simulink model "ControlLineal"  (R2024a)
settings: Solver=ode4  StartTime=0.0  StopTime=20  FixedStep=.01  MinStep=.01  RelTol=1e-3
settings Model: Creator=YTLATELPO  LastModifiedBy=alegaco
settings RTWCC: GPUComputeCapability=3.5

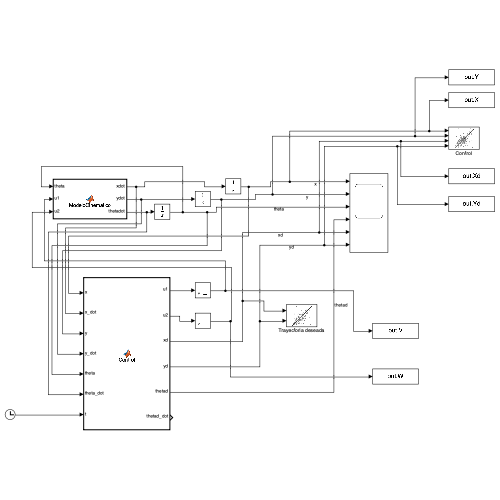
[thumbnail: Simulink's stored preview of the top-level diagram]
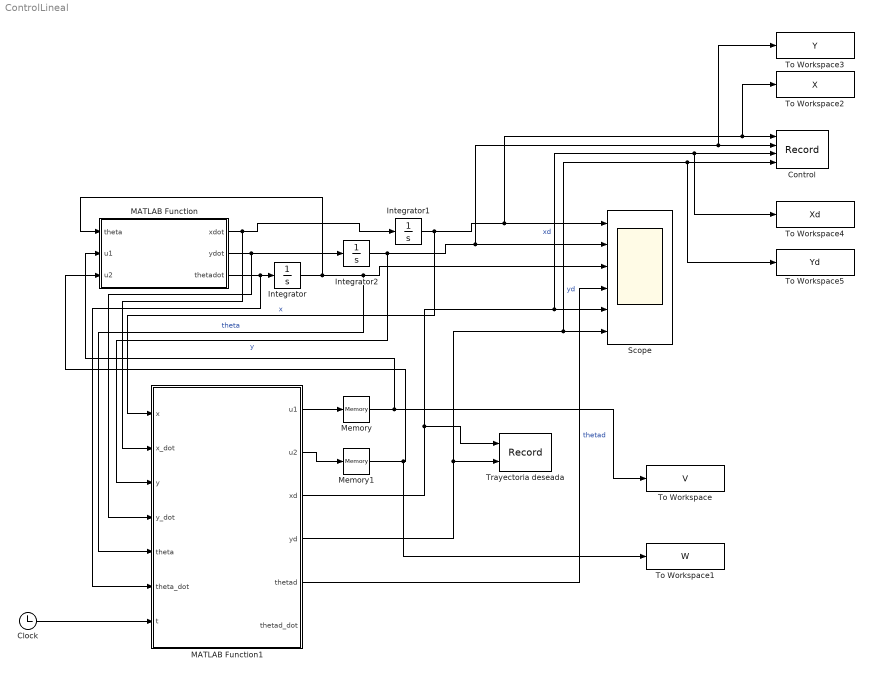
== system ControlLineal ==
  Clock : Clock
  Control : Record  FileSettingsInternal="{\"entries\":[{\"content\":{\"excelSettings\":{\"content\":{},\"type\":\"Streamout.ExcelSettings\"}},\"type\":\"Streamout.FileSettingStorage\",\"uuid\":\"\"}],\"packageUris\":[\"http:\\/\\/schema.mathworks.com\\/mf0\\/streamout_blocks\\/R2020a\"],\"version\":\"1.0\"}"  Layout=[1 1]  SignalsInternal="{\"entries\":[{\"content\":{\"signals\":[{\"content\":{\"blockPath\":[],\"dimensions\":[1],\"domain\":\"\",\"lineColor\":\"#139fff\",\"lineWidth\":4,\"plots\":[ 1 ],\"port\":1,\"sid\":[\"\"],\"signalID\":1,\"signalName\":\"x\"},\"type\":\"RecordBlkView.Signal\",\"uuid\":\"\"},{\"content\":{\"blockPath\":[],\"dimensions\":[1],\"domain\":\"\",\"lineColor\":\"#139fff\",\"lineWidth\":4,\"plots\":[ 1 ],\"port\":2,\"sid\":[\"\"],\"signalID\":2,\"signalName\":\"y\"},\"type\":\"RecordBlkView.Signal\",\"uuid\":\"\"},{\"content\":{\"blockPath\":[],\"dimensions\":[1],\"domain\":\"\",\"lineColor\":\"#ff6929\",\"lineStyle\":\"DASHED\",\"lineWidth\":4,\"plots\":[ 1 ],\"port\":3,\"sid\":[\"\"],\"signalID\":3,\"signalName\":\"xd\"},\"type\":\"RecordBlkView.Signal\",\"uuid\":\"\"},{\"content\":{\"blockPath\":[],\"dimensions\":[1],\"domain\":\"\",\"lineColor\":\"#ff6929\",\"lineStyle\":\"DASHED\",\"lineWidth\":4,\"plots\":[ 1 ],\"port\":4,\"sid\":[\"\"],\"signalID\":4,\"signalName\":\"yd\"},\"type\":\"RecordBlkView.Signal\",\"uuid\":\"\"}]},\"type\":\"RecordBlkView.InputSignals\",\"uuid\":\"\"}],\"packageUris\":[\"http:\\/\\/schema.mathworks.com\\/mf0\\/streamout_blocks\\/R2020a\"],\"version\":\"1.0\"}"  VisualizationBindings="{\"xyplotplugin\":{\"info\":[{\"series\":[{\"bindingParametersList\":[{\"parameter\":\"X-Axis\",\"signalID\":1,\"signalName\":\"x\"},{\"parameter\":\"Y-Axis\",\"signalID\":2,\"signalName\":\"y\"}],\"seriesID\":0},{\"bindingParametersList\":[{\"parameter\":\"X-Axis\",\"signalID\":3,\"signalName\":\"xd\"},{\"parameter\":\"Y-Axis\",\"signalID\":4,\"signalName\":\"yd\"}],\"seriesID\":1}],\"subplotID\":1}]}}"  CompatibilityTag=XY
  Integrator : Integrator
  Integrator1 : Integrator  InitialCondition=2
  Integrator2 : Integrator
  MATLAB Function : MATLAB Function  TreatAsAtomicUnit=on
  MATLAB Function1 : MATLAB Function  TreatAsAtomicUnit=on
  Memory : Memory
  Memory1 : Memory
  Scope : Scope  NumInputPorts=6
  To Workspace : ToWorkspace  VariableName=V  SampleTime=-1
  To Workspace1 : ToWorkspace  VariableName=W  SampleTime=-1
  To Workspace2 : ToWorkspace  VariableName=X  SampleTime=-1
  To Workspace3 : ToWorkspace  VariableName=Y  SampleTime=-1
  To Workspace4 : ToWorkspace  VariableName=Xd  SampleTime=-1
  To Workspace5 : ToWorkspace  VariableName=Yd  SampleTime=-1
  Trayectoria deseada : Record  FileSettingsInternal="{\"entries\":[{\"content\":{\"excelSettings\":{\"content\":{},\"type\":\"Streamout.ExcelSettings\"}},\"type\":\"Streamout.FileSettingStorage\",\"uuid\":\"\"}],\"packageUris\":[\"http:\\/\\/schema.mathworks.com\\/mf0\\/streamout_blocks\\/R2020a\"],\"version\":\"1.0\"}"  Layout=[1 1]  SignalsInternal="{\"entries\":[{\"content\":{\"signals\":[{\"content\":{\"blockPath\":[],\"dimensions\":[1],\"domain\":\"\",\"lineColor\":\"#139fff\",\"lineWidth\":5,\"plots\":[ 1 ],\"port\":1,\"sid\":[\"\"],\"signalID\":1,\"signalName\":\"xd\"},\"type\":\"RecordBlkView.Signal\",\"uuid\":\"\"},{\"content\":{\"blockPath\":[],\"dimensions\":[1],\"domain\":\"\",\"lineColor\":\"#139fff\",\"lineWidth\":5,\"plots\":[ 1 ],\"port\":2,\"sid\":[\"\"],\"signalID\":2,\"signalName\":\"yd\"},\"type\":\"RecordBlkView.Signal\",\"uuid\":\"\"}]},\"type\":\"RecordBlkView.InputSignals\",\"uuid\":\"\"}],\"packageUris\":[\"http:\\/\\/schema.mathworks.com\\/mf0\\/streamout_blocks\\/R2020a\"],\"version\":\"1.0\"}"  VisualizationBindings="{\"sparklinesplugin\":{\"info\":[{\"bindingParametersList\":[],\"subplotID\":2}]},\"xyplotplugin\":{\"info\":[{\"series\":[{\"bindingParametersList\":[{\"parameter\":\"X-Axis\",\"signalID\":1,\"signalName\":\"xd\"},{\"parameter\":\"Y-Axis\",\"signalID\":2,\"signalName\":\"yd\"}],\"seriesID\":0}],\"subplotID\":1}]}}"  CompatibilityTag=XY
  wires:
  MATLAB Function/3(thetadot) -> MATLAB Function1/6(theta_dot), Integrator/1
  Integrator1/1 -> MATLAB Function1/1(x), To Workspace2/1, Control/1, Scope/1  "x"
  Integrator2/1 -> MATLAB Function1/3(y), To Workspace3/1, Control/2, Scope/2  "y"
  Clock/1 -> MATLAB Function1/7(t)
  MATLAB Function1/1(u1) -> Memory/1
  MATLAB Function1/2(u2) -> Memory1/1
  Memory/1 -> To Workspace/1, MATLAB Function/2(u1)
  Memory1/1 -> To Workspace1/1, MATLAB Function/3(u2)
  Integrator/1 -> MATLAB Function/1(theta), MATLAB Function1/5(theta), Scope/3  "theta"
  MATLAB Function1/3(xd) -> To Workspace4/1, Control/3, Scope/5, Trayectoria deseada/1  "xd"
  MATLAB Function1/4(yd) -> To Workspace5/1, Control/4, Scope/6, Trayectoria deseada/2  "yd"
  MATLAB Function1/5(thetad) -> Scope/4  "thetad"
  MATLAB Function/1(xdot) -> MATLAB Function1/2(x_dot), Integrator1/1
  MATLAB Function/2(ydot) -> MATLAB Function1/4(y_dot), Integrator2/1

== matlab function ControlLineal/MATLAB Function1 ==
  data: x input; x_dot input; y input; y_dot input; theta input; theta_dot input; u1 output; u2 output; t input; xd output; yd output; thetad output; thetad_dot output
function [u1,u2,xd,yd,thetad,thetad_dot] = Control(x,x_dot,y,y_dot,theta,theta_dot,t)
k1=1;
k2=1;
k3=1.5;

xd = 2.8;
yd = 0.3;
thetad = 0;
thetad_dot=0;
u1 = 0;
u2 = 0;

if t > 4
    xd = 2.8;
    xd_dot = 0;

    yd = 0.3+(t-4)/2;
    yd_dot = 1/2;

    if yd > 4
        yd = 4;
        yd_dot = 0;
    end

    thetad = pi / 2;
    thetad_dot = 0;

    u1 = (xd_dot - k1*(x-xd))*cos(theta) + (yd_dot-k2*(y-yd))*sin(theta);
    u2 = thetad_dot-k3*sin(theta-thetad);
end

== matlab function ControlLineal/MATLAB Function ==
  data: theta input; xdot output; u1 input; u2 input; ydot output; thetadot output
function [xdot,ydot,thetadot] = ModeloCinematico(theta,u1,u2)

xdot = u1*cos(theta);
ydot = u1*sin(theta);
thetadot = u2;
